simulink library "combinedController"  (R2018b)
settings: Solver=VariableStepAuto  StartTime=0.0  StopTime=10.0  RelTol=1e-3
libraries: pathFollowingController_cl x1
settings Model: Creator=jldanie5  LastModifiedBy=jldanie5

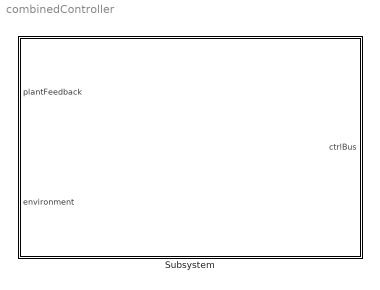
== system combinedController ==
  Subsystem : Subsystem

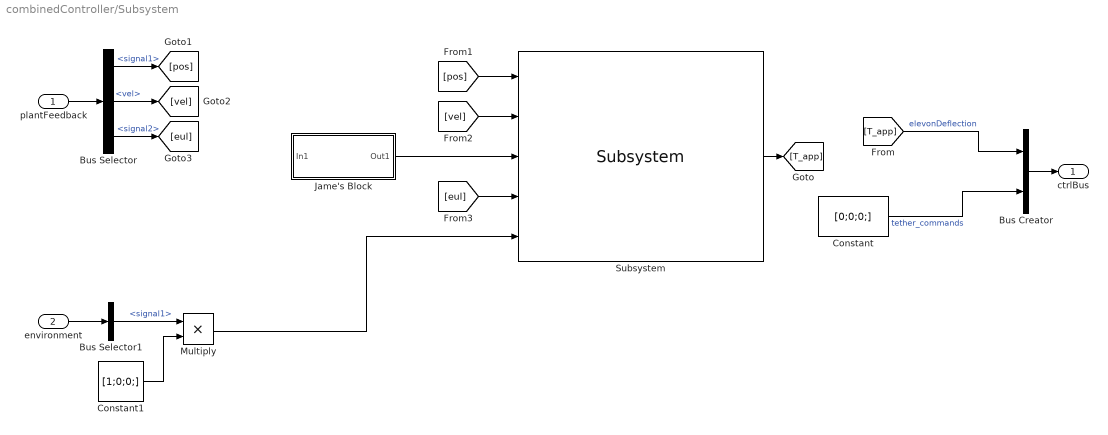
== system combinedController/Subsystem ==
  plantFeedback : Inport
  environment : Inport  Port=2
  Bus Creator : BusCreator  Inputs=2
  Bus Selector : BusSelector  OutputSignals=signal1,vel,signal2
  Bus Selector1 : BusSelector  OutputSignals=signal1
  Constant : Constant  Value=[0;0;0;]
  Constant1 : Constant  Value=[1;0;0;]
  Jame's Block : Subsystem
  Multiply : Product
  Subsystem : pathFollowingController_cl/Subsystem  AoA_des=0  controlMat=0  ctrlSigMax=0
  ctrlBus : Outport
  wires:
  Subsystem/1 -> [T_app]
  Constant1/1 -> Multiply/2
  Multiply/1 -> Subsystem/5
  Jame's Block/1(Out1) -> Subsystem/3
  Bus Creator/1 -> ctrlBus/1
  Constant/1 -> Bus Creator/2  "tether_commands"
  [T_app] -> Bus Creator/1  "elevonDeflection"
  Bus Selector1/1 -> Multiply/1  "<signal1>"
  environment/1 -> Bus Selector1/1
  plantFeedback/1 -> Bus Selector/1
  Bus Selector/2 -> [vel]  "<vel>"
  Bus Selector/1 -> [pos]  "<signal1>"
  Bus Selector/3 -> [eul]  "<signal2>"
  [pos] -> Subsystem/1
  [vel] -> Subsystem/2
  [eul] -> Subsystem/4

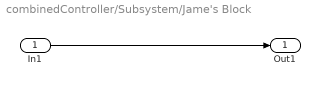
== system combinedController/Subsystem/Jame's Block ==
  In1 : Inport
  Out1 : Outport
  wires:
  In1/1 -> Out1/1
